simulink model "DuoCopter1"  (R2015b)
settings: Solver=FixedStepAuto  StartTime=0.0  StopTime=150  FixedStep=.01  MaxStep=10  RelTol=1e-3
values from neighbouring files (symbols this model uses):
  AoAMax = 18    [MainDataFile.m]
  RodMass = 1505    [MainDataFile.m]
  s = saveObjectImpl@matlab.System(obj)    [moving_average.m]
undefined symbols (not defined in the file or in its folder): X, Y, Z
libraries: sm_lib x35, Library_Octocopter x19, nesl_utility x17, simulink x3, dspfdesign x1, aerolibfltsims x1
(part 2 of 2)

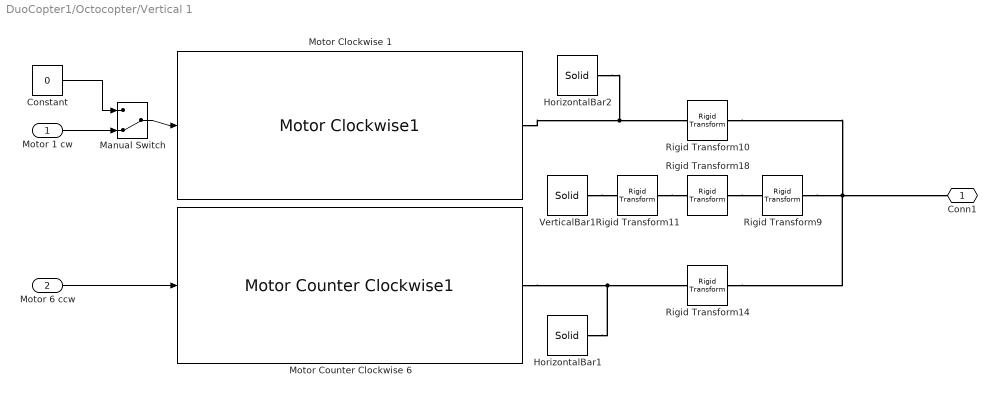
== system DuoCopter1/Octocopter/Vertical 1 ==
  Motor 1 cw : Inport
  Motor 6 ccw : Inport  Port=2
  Constant : Constant  Value=0
  HorizontalBar1 : sm_lib/Body Elements/Solid  InertiaType=PointMass  Mass=462.5  MassUnits=kg  CenterOfMass=[0 0 0]  CenterOfMassUnits=m  MomentsOfInertia=[1 1 1]  MomentsOfInertiaUnits=kg*m^2  ProductsOfInertia=[0 0 0]  ProductsOfInertiaUnits=kg*m^2  DensityBased=on  Density=DensityTube  DensityUnits=kg/(m^3)  DoExposeReferenceFrame=on  SerializedFrames=<Frames/>  GraphicType=FromGeometry  MarkerShape=Sphere  MarkerSize=10  MarkerSizeUnits=m  GraphicVisPropType=SimpleVisualProperties  GraphicDiffuseColor=[0.5 0.5 0.5]  GraphicSpecularColor=[0.5 0.5 0.5 1.0]  GraphicAmbientColor=[0.15 0.15 0.15 1.0]  GraphicEmissiveColor=[0.0 0.0 0.0 1.0]  GraphicShininess=75  GraphicOpacity=1.0  GeometryShape=Sphere  RectangleSize=[1 1]  RectangleSizeUnits=m  BrickDimensions=[1 1 1]  BrickDimensionUnits=m  CylinderRadius=RadiusTube  CylinderRadiusUnits=m  CylinderLength=RodLength  CylinderLengthUnits=m  SphereRadius=.5  SphereRadiusUnits=m  EllipsoidRadii=[1 1 1]  EllipsoidRadiiUnits=m  ExtrusionCrossSection=[1 1; -1 1; -1 -1; 1 -1]  ExtrusionCrossSectionUnits=m  ExtrusionLength=1  ExtrusionLengthUnits=m  PolygonNumSides=3  PolygonOuterRadius=1  PolygonOuterRadiusUnits=m  ExtGeomFileType=STL  ExtGeomFileUnits=m  RevolutionCrossSection=[1 1; 1 -1; 2 -1; 2 1]  RevolutionCrossSectionUnits=m  RevolutionExtent=Full  RevolutionAngle=180  RevolutionAngleUnits=deg  BlockFunction=simmechanics.library.body_elements.solid
  HorizontalBar2 : sm_lib/Body Elements/Solid  InertiaType=PointMass  Mass=462.5  MassUnits=kg  CenterOfMass=[0 0 0]  CenterOfMassUnits=m  MomentsOfInertia=[1 1 1]  MomentsOfInertiaUnits=kg*m^2  ProductsOfInertia=[0 0 0]  ProductsOfInertiaUnits=kg*m^2  DensityBased=on  Density=DensityTube  DensityUnits=kg/(m^3)  DoExposeReferenceFrame=on  SerializedFrames=<Frames/>  GraphicType=FromGeometry  MarkerShape=Sphere  MarkerSize=10  MarkerSizeUnits=m  GraphicVisPropType=SimpleVisualProperties  GraphicDiffuseColor=[0.5 0.5 0.5]  GraphicSpecularColor=[0.5 0.5 0.5 1.0]  GraphicAmbientColor=[0.15 0.15 0.15 1.0]  GraphicEmissiveColor=[0.0 0.0 0.0 1.0]  GraphicShininess=75  GraphicOpacity=1.0  GeometryShape=Sphere  RectangleSize=[1 1]  RectangleSizeUnits=m  BrickDimensions=[1 1 1]  BrickDimensionUnits=m  CylinderRadius=RadiusTube  CylinderRadiusUnits=m  CylinderLength=RodLength  CylinderLengthUnits=m  SphereRadius=.5  SphereRadiusUnits=m  EllipsoidRadii=[1 1 1]  EllipsoidRadiiUnits=m  ExtrusionCrossSection=[1 1; -1 1; -1 -1; 1 -1]  ExtrusionCrossSectionUnits=m  ExtrusionLength=1  ExtrusionLengthUnits=m  PolygonNumSides=3  PolygonOuterRadius=1  PolygonOuterRadiusUnits=m  ExtGeomFileType=STL  ExtGeomFileUnits=m  RevolutionCrossSection=[1 1; 1 -1; 2 -1; 2 1]  RevolutionCrossSectionUnits=m  RevolutionExtent=Full  RevolutionAngle=180  RevolutionAngleUnits=deg  BlockFunction=simmechanics.library.body_elements.solid
  Manual Switch : ManualSwitch  CurrentSetting=0
  Motor Clockwise 1 : Library_Octocopter/Motor Clockwise1
  Motor Counter Clockwise 6 : Library_Octocopter/Motor Counter Clockwise1
  Rigid Transform10 : sm_lib/Frames and Transforms/Rigid Transform  TranslationMethod=Cartesian  TranslationLengthUnit=m  TranslationStandardAxis=+Z  TranslationStandardOffset=0  TranslationCartesianOffset=PositionEngine1  TranslationROffset=0  TranslationROffsetUnits=m  TranslationZOffset=0  TranslationZOffsetUnits=m  TranslationThetaOffset=0  TranslationThetaOffsetUnits=deg  RotationMethod=None  RotationAngleUnits=deg  RotationStandardAxis=+Z  RotationAngle=0  RotationArbitraryAxis=[0 0 1]  FollAlignAxisA=+X  BaseAlignAxisA=+Y  FollAlignAxisB=+Y  BaseAlignAxisB=+Z  RotationSequenceAxes=FollowerAxes  RotationSequence=XYX  RotationSequenceAngles=[0 0 0]  RotationSequenceAnglesUnits=deg  RotationMatrix=[1 0 0; 0 1 0; 0 0 1]  BlockFunction=simmechanics.library.frames_transforms.rigid_transform
  Rigid Transform11 : sm_lib/Frames and Transforms/Rigid Transform  TranslationMethod=Cartesian  TranslationLengthUnit=m  TranslationStandardAxis=+Z  TranslationStandardOffset=0  TranslationCartesianOffset=[0 0 0]  TranslationROffset=0  TranslationROffsetUnits=m  TranslationZOffset=0  TranslationZOffsetUnits=m  TranslationThetaOffset=0  TranslationThetaOffsetUnits=deg  RotationMethod=StandardAxis  RotationAngleUnits=deg  RotationStandardAxis=+Y  RotationAngle=90  RotationArbitraryAxis=[0 0 1]  FollAlignAxisA=+X  BaseAlignAxisA=+Y  FollAlignAxisB=+Y  BaseAlignAxisB=+Z  RotationSequenceAxes=FollowerAxes  RotationSequence=XYX  RotationSequenceAngles=[0 0 0]  RotationSequenceAnglesUnits=deg  RotationMatrix=[1 0 0; 0 1 0; 0 0 1]  BlockFunction=simmechanics.library.frames_transforms.rigid_transform
  Rigid Transform14 : sm_lib/Frames and Transforms/Rigid Transform  TranslationMethod=Cartesian  TranslationLengthUnit=m  TranslationStandardAxis=+Z  TranslationStandardOffset=0  TranslationCartesianOffset=PositionEngine6  TranslationROffset=0  TranslationROffsetUnits=m  TranslationZOffset=0  TranslationZOffsetUnits=m  TranslationThetaOffset=0  TranslationThetaOffsetUnits=deg  RotationMethod=None  RotationAngleUnits=deg  RotationStandardAxis=+Z  RotationAngle=0  RotationArbitraryAxis=[0 0 1]  FollAlignAxisA=+X  BaseAlignAxisA=+Y  FollAlignAxisB=+Y  BaseAlignAxisB=+Z  RotationSequenceAxes=FollowerAxes  RotationSequence=XYX  RotationSequenceAngles=[0 0 0]  RotationSequenceAnglesUnits=deg  RotationMatrix=[1 0 0; 0 1 0; 0 0 1]  BlockFunction=simmechanics.library.frames_transforms.rigid_transform
  Rigid Transform18 : sm_lib/Frames and Transforms/Rigid Transform  TranslationMethod=None  TranslationLengthUnit=m  TranslationStandardAxis=+Z  TranslationStandardOffset=0  TranslationCartesianOffset=[0 0 0]  TranslationROffset=0  TranslationROffsetUnits=m  TranslationZOffset=0  TranslationZOffsetUnits=m  TranslationThetaOffset=0  TranslationThetaOffsetUnits=deg  RotationMethod=StandardAxis  RotationAngleUnits=deg  RotationStandardAxis=+Z  RotationAngle=90  RotationArbitraryAxis=[0 0 1]  FollAlignAxisA=+X  BaseAlignAxisA=+Y  FollAlignAxisB=+Y  BaseAlignAxisB=+Z  RotationSequenceAxes=FollowerAxes  RotationSequence=XYX  RotationSequenceAngles=[0 0 0]  RotationSequenceAnglesUnits=deg  RotationMatrix=[1 0 0; 0 1 0; 0 0 1]  BlockFunction=simmechanics.library.frames_transforms.rigid_transform
  Rigid Transform9 : sm_lib/Frames and Transforms/Rigid Transform  TranslationMethod=Cartesian  TranslationLengthUnit=m  TranslationStandardAxis=+Z  TranslationStandardOffset=0  TranslationCartesianOffset=VerticalBar1  TranslationROffset=0  TranslationROffsetUnits=m  TranslationZOffset=0  TranslationZOffsetUnits=m  TranslationThetaOffset=0  TranslationThetaOffsetUnits=deg  RotationMethod=None  RotationAngleUnits=deg  RotationStandardAxis=+Z  RotationAngle=0  RotationArbitraryAxis=[0 0 1]  FollAlignAxisA=+X  BaseAlignAxisA=+Y  FollAlignAxisB=+Y  BaseAlignAxisB=+Z  RotationSequenceAxes=FollowerAxes  RotationSequence=XYX  RotationSequenceAngles=[0 0 0]  RotationSequenceAnglesUnits=deg  RotationMatrix=[1 0 0; 0 1 0; 0 0 1]  BlockFunction=simmechanics.library.frames_transforms.rigid_transform
  VerticalBar1 : sm_lib/Body Elements/Solid  InertiaType=CalculateFromGeometry  Mass=RodMass  MassUnits=kg  CenterOfMass=[0 0 0]  CenterOfMassUnits=m  MomentsOfInertia=[1 1 1]  MomentsOfInertiaUnits=kg*m^2  ProductsOfInertia=[0 0 0]  ProductsOfInertiaUnits=kg*m^2  DensityBased=off  Density=DensityTube  DensityUnits=kg/(m^3)  DoExposeReferenceFrame=on  SerializedFrames=<Frames/>  GraphicType=FromGeometry  MarkerShape=Sphere  MarkerSize=10  MarkerSizeUnits=m  GraphicVisPropType=SimpleVisualProperties  GraphicDiffuseColor=[0.5 0.5 0.5]  GraphicSpecularColor=[0.5 0.5 0.5 1.0]  GraphicAmbientColor=[0.15 0.15 0.15 1.0]  GraphicEmissiveColor=[0.0 0.0 0.0 1.0]  GraphicShininess=75  GraphicOpacity=1.0  GeometryShape=Cylinder  RectangleSize=[1 1]  RectangleSizeUnits=m  BrickDimensions=[1 1 1]  BrickDimensionUnits=m  CylinderRadius=RadiusTube  CylinderRadiusUnits=m  CylinderLength=RodLength  CylinderLengthUnits=m  SphereRadius=1  SphereRadiusUnits=m  EllipsoidRadii=[1 1 1]  EllipsoidRadiiUnits=m  ExtrusionCrossSection=[1 1; -1 1; -1 -1; 1 -1]  ExtrusionCrossSectionUnits=m  ExtrusionLength=1  ExtrusionLengthUnits=m  PolygonNumSides=3  PolygonOuterRadius=1  PolygonOuterRadiusUnits=m  ExtGeomFileType=STL  ExtGeomFileUnits=m  RevolutionCrossSection=[1 1; 1 -1; 2 -1; 2 1]  RevolutionCrossSectionUnits=m  RevolutionExtent=Full  RevolutionAngle=180  RevolutionAngleUnits=deg  BlockFunction=simmechanics.library.body_elements.solid
  Conn1 : PMIOPort  Port=1  Side=Right
  wires:
  Motor 6 ccw/1 -> Motor Counter Clockwise 6/1
  Constant/1 -> Manual Switch/1
  Motor 1 cw/1 -> Manual Switch/2
  Manual Switch/1 -> Motor Clockwise 1/1
  connections:
  VerticalBar1/RConn1 -- Rigid Transform11/RConn1
  Rigid Transform14/LConn1 -- Conn1/RConn1 -- Rigid Transform10/LConn1 -- Rigid Transform9/LConn1
  Motor Counter Clockwise 6/RConn1 -- HorizontalBar1/RConn1 -- Rigid Transform14/RConn1
  Motor Clockwise 1/RConn1 -- HorizontalBar2/RConn1 -- Rigid Transform10/RConn1
  Rigid Transform11/LConn1 -- Rigid Transform18/RConn1
  Rigid Transform18/LConn1 -- Rigid Transform9/RConn1

== system DuoCopter1/Octocopter/Vertical 2 ==
  "Motor 2 ccw " : Inport
  Motor 5 cw : Inport  Port=2
  HorizontalBar1 : sm_lib/Body Elements/Solid  InertiaType=PointMass  Mass=462.5  MassUnits=kg  CenterOfMass=[0 0 0]  CenterOfMassUnits=m  MomentsOfInertia=[1 1 1]  MomentsOfInertiaUnits=kg*m^2  ProductsOfInertia=[0 0 0]  ProductsOfInertiaUnits=kg*m^2  DensityBased=on  Density=DensityTube  DensityUnits=kg/(m^3)  DoExposeReferenceFrame=on  SerializedFrames=<Frames/>  GraphicType=FromGeometry  MarkerShape=Sphere  MarkerSize=10  MarkerSizeUnits=m  GraphicVisPropType=SimpleVisualProperties  GraphicDiffuseColor=[0.5 0.5 0.5]  GraphicSpecularColor=[0.5 0.5 0.5 1.0]  GraphicAmbientColor=[0.15 0.15 0.15 1.0]  GraphicEmissiveColor=[0.0 0.0 0.0 1.0]  GraphicShininess=75  GraphicOpacity=1.0  GeometryShape=Sphere  RectangleSize=[1 1]  RectangleSizeUnits=m  BrickDimensions=[1 1 1]  BrickDimensionUnits=m  CylinderRadius=RadiusTube  CylinderRadiusUnits=m  CylinderLength=RodLength  CylinderLengthUnits=m  SphereRadius=.5  SphereRadiusUnits=m  EllipsoidRadii=[1 1 1]  EllipsoidRadiiUnits=m  ExtrusionCrossSection=[1 1; -1 1; -1 -1; 1 -1]  ExtrusionCrossSectionUnits=m  ExtrusionLength=1  ExtrusionLengthUnits=m  PolygonNumSides=3  PolygonOuterRadius=1  PolygonOuterRadiusUnits=m  ExtGeomFileType=STL  ExtGeomFileUnits=m  RevolutionCrossSection=[1 1; 1 -1; 2 -1; 2 1]  RevolutionCrossSectionUnits=m  RevolutionExtent=Full  RevolutionAngle=180  RevolutionAngleUnits=deg  BlockFunction=simmechanics.library.body_elements.solid
  HorizontalBar2 : sm_lib/Body Elements/Solid  InertiaType=PointMass  Mass=462.5  MassUnits=kg  CenterOfMass=[0 0 0]  CenterOfMassUnits=m  MomentsOfInertia=[1 1 1]  MomentsOfInertiaUnits=kg*m^2  ProductsOfInertia=[0 0 0]  ProductsOfInertiaUnits=kg*m^2  DensityBased=on  Density=DensityTube  DensityUnits=kg/(m^3)  DoExposeReferenceFrame=on  SerializedFrames=<Frames/>  GraphicType=FromGeometry  MarkerShape=Sphere  MarkerSize=10  MarkerSizeUnits=m  GraphicVisPropType=SimpleVisualProperties  GraphicDiffuseColor=[0.5 0.5 0.5]  GraphicSpecularColor=[0.5 0.5 0.5 1.0]  GraphicAmbientColor=[0.15 0.15 0.15 1.0]  GraphicEmissiveColor=[0.0 0.0 0.0 1.0]  GraphicShininess=75  GraphicOpacity=1.0  GeometryShape=Sphere  RectangleSize=[1 1]  RectangleSizeUnits=m  BrickDimensions=[1 1 1]  BrickDimensionUnits=m  CylinderRadius=RadiusTube  CylinderRadiusUnits=m  CylinderLength=RodLength  CylinderLengthUnits=m  SphereRadius=.5  SphereRadiusUnits=m  EllipsoidRadii=[1 1 1]  EllipsoidRadiiUnits=m  ExtrusionCrossSection=[1 1; -1 1; -1 -1; 1 -1]  ExtrusionCrossSectionUnits=m  ExtrusionLength=1  ExtrusionLengthUnits=m  PolygonNumSides=3  PolygonOuterRadius=1  PolygonOuterRadiusUnits=m  ExtGeomFileType=STL  ExtGeomFileUnits=m  RevolutionCrossSection=[1 1; 1 -1; 2 -1; 2 1]  RevolutionCrossSectionUnits=m  RevolutionExtent=Full  RevolutionAngle=180  RevolutionAngleUnits=deg  BlockFunction=simmechanics.library.body_elements.solid
  Motor Clockwise 5 : Library_Octocopter/Motor Clockwise1
  Motor Counter Clockwise 2 : Library_Octocopter/Motor Counter Clockwise1
  Rigid Transform12 : sm_lib/Frames and Transforms/Rigid Transform  TranslationMethod=Cartesian  TranslationLengthUnit=m  TranslationStandardAxis=+Z  TranslationStandardOffset=0  TranslationCartesianOffset=VerticalBar2  TranslationROffset=0  TranslationROffsetUnits=m  TranslationZOffset=0  TranslationZOffsetUnits=m  TranslationThetaOffset=0  TranslationThetaOffsetUnits=deg  RotationMethod=None  RotationAngleUnits=deg  RotationStandardAxis=+Z  RotationAngle=0  RotationArbitraryAxis=[0 0 1]  FollAlignAxisA=+X  BaseAlignAxisA=+Y  FollAlignAxisB=+Y  BaseAlignAxisB=+Z  RotationSequenceAxes=FollowerAxes  RotationSequence=XYX  RotationSequenceAngles=[0 0 0]  RotationSequenceAnglesUnits=deg  RotationMatrix=[1 0 0; 0 1 0; 0 0 1]  BlockFunction=simmechanics.library.frames_transforms.rigid_transform
  Rigid Transform13 : sm_lib/Frames and Transforms/Rigid Transform  TranslationMethod=Cartesian  TranslationLengthUnit=m  TranslationStandardAxis=+Z  TranslationStandardOffset=0  TranslationCartesianOffset=PositionEngine2  TranslationROffset=0  TranslationROffsetUnits=m  TranslationZOffset=0  TranslationZOffsetUnits=m  TranslationThetaOffset=0  TranslationThetaOffsetUnits=deg  RotationMethod=None  RotationAngleUnits=deg  RotationStandardAxis=+Z  RotationAngle=0  RotationArbitraryAxis=[0 0 1]  FollAlignAxisA=+X  BaseAlignAxisA=+Y  FollAlignAxisB=+Y  BaseAlignAxisB=+Z  RotationSequenceAxes=FollowerAxes  RotationSequence=XYX  RotationSequenceAngles=[0 0 0]  RotationSequenceAnglesUnits=deg  RotationMatrix=[1 0 0; 0 1 0; 0 0 1]  BlockFunction=simmechanics.library.frames_transforms.rigid_transform
  Rigid Transform15 : sm_lib/Frames and Transforms/Rigid Transform  TranslationMethod=Cartesian  TranslationLengthUnit=m  TranslationStandardAxis=+Z  TranslationStandardOffset=0  TranslationCartesianOffset=[0 0 0]  TranslationROffset=0  TranslationROffsetUnits=m  TranslationZOffset=0  TranslationZOffsetUnits=m  TranslationThetaOffset=0  TranslationThetaOffsetUnits=deg  RotationMethod=StandardAxis  RotationAngleUnits=deg  RotationStandardAxis=+Y  RotationAngle=90  RotationArbitraryAxis=[0 0 1]  FollAlignAxisA=+X  BaseAlignAxisA=+Y  FollAlignAxisB=+Y  BaseAlignAxisB=+Z  RotationSequenceAxes=FollowerAxes  RotationSequence=XYX  RotationSequenceAngles=[0 0 0]  RotationSequenceAnglesUnits=deg  RotationMatrix=[1 0 0; 0 1 0; 0 0 1]  BlockFunction=simmechanics.library.frames_transforms.rigid_transform
  Rigid Transform16 : sm_lib/Frames and Transforms/Rigid Transform  TranslationMethod=Cartesian  TranslationLengthUnit=m  TranslationStandardAxis=+Z  TranslationStandardOffset=0  TranslationCartesianOffset=PositionEngine5  TranslationROffset=0  TranslationROffsetUnits=m  TranslationZOffset=0  TranslationZOffsetUnits=m  TranslationThetaOffset=0  TranslationThetaOffsetUnits=deg  RotationMethod=None  RotationAngleUnits=deg  RotationStandardAxis=+Z  RotationAngle=0  RotationArbitraryAxis=[0 0 1]  FollAlignAxisA=+X  BaseAlignAxisA=+Y  FollAlignAxisB=+Y  BaseAlignAxisB=+Z  RotationSequenceAxes=FollowerAxes  RotationSequence=XYX  RotationSequenceAngles=[0 0 0]  RotationSequenceAnglesUnits=deg  RotationMatrix=[1 0 0; 0 1 0; 0 0 1]  BlockFunction=simmechanics.library.frames_transforms.rigid_transform
  Rigid Transform17 : sm_lib/Frames and Transforms/Rigid Transform  TranslationMethod=None  TranslationLengthUnit=m  TranslationStandardAxis=+Z  TranslationStandardOffset=0  TranslationCartesianOffset=[0 0 0]  TranslationROffset=0  TranslationROffsetUnits=m  TranslationZOffset=0  TranslationZOffsetUnits=m  TranslationThetaOffset=0  TranslationThetaOffsetUnits=deg  RotationMethod=StandardAxis  RotationAngleUnits=deg  RotationStandardAxis=+Z  RotationAngle=90  RotationArbitraryAxis=[0 0 1]  FollAlignAxisA=+X  BaseAlignAxisA=+Y  FollAlignAxisB=+Y  BaseAlignAxisB=+Z  RotationSequenceAxes=FollowerAxes  RotationSequence=XYX  RotationSequenceAngles=[0 0 0]  RotationSequenceAnglesUnits=deg  RotationMatrix=[1 0 0; 0 1 0; 0 0 1]  BlockFunction=simmechanics.library.frames_transforms.rigid_transform
  VerticalBar 2 : sm_lib/Body Elements/Solid  InertiaType=CalculateFromGeometry  Mass=RodMass  MassUnits=kg  CenterOfMass=[0 0 0]  CenterOfMassUnits=m  MomentsOfInertia=[1 1 1]  MomentsOfInertiaUnits=kg*m^2  ProductsOfInertia=[0 0 0]  ProductsOfInertiaUnits=kg*m^2  DensityBased=off  Density=DensityTube  DensityUnits=kg/(m^3)  DoExposeReferenceFrame=on  SerializedFrames=<Frames/>  GraphicType=FromGeometry  MarkerShape=Sphere  MarkerSize=10  MarkerSizeUnits=m  GraphicVisPropType=SimpleVisualProperties  GraphicDiffuseColor=[0.5 0.5 0.5]  GraphicSpecularColor=[0.5 0.5 0.5 1.0]  GraphicAmbientColor=[0.15 0.15 0.15 1.0]  GraphicEmissiveColor=[0.0 0.0 0.0 1.0]  GraphicShininess=75  GraphicOpacity=1.0  GeometryShape=Cylinder  RectangleSize=[1 1]  RectangleSizeUnits=m  BrickDimensions=[1 1 1]  BrickDimensionUnits=m  CylinderRadius=RadiusTube  CylinderRadiusUnits=m  CylinderLength=RodLength  CylinderLengthUnits=m  SphereRadius=1  SphereRadiusUnits=m  EllipsoidRadii=[1 1 1]  EllipsoidRadiiUnits=m  ExtrusionCrossSection=[1 1; -1 1; -1 -1; 1 -1]  ExtrusionCrossSectionUnits=m  ExtrusionLength=1  ExtrusionLengthUnits=m  PolygonNumSides=3  PolygonOuterRadius=1  PolygonOuterRadiusUnits=m  ExtGeomFileType=STL  ExtGeomFileUnits=m  RevolutionCrossSection=[1 1; 1 -1; 2 -1; 2 1]  RevolutionCrossSectionUnits=m  RevolutionExtent=Full  RevolutionAngle=180  RevolutionAngleUnits=deg  BlockFunction=simmechanics.library.body_elements.solid
  Conn1 : PMIOPort  Port=1  Side=Right
  wires:
  Motor 5 cw/1 -> Motor Clockwise 5/1
  "Motor 2 ccw "/1 -> Motor Counter Clockwise 2/1
  connections:
  VerticalBar 2/RConn1 -- Rigid Transform15/RConn1
  Rigid Transform17/RConn1 -- Rigid Transform15/LConn1
  Rigid Transform17/LConn1 -- Rigid Transform12/RConn1
  Rigid Transform16/LConn1 -- Conn1/RConn1 -- Rigid Transform13/LConn1 -- Rigid Transform12/LConn1
  Motor Counter Clockwise 2/RConn1 -- HorizontalBar2/RConn1 -- Rigid Transform13/RConn1
  Motor Clockwise 5/RConn1 -- HorizontalBar1/RConn1 -- Rigid Transform16/RConn1

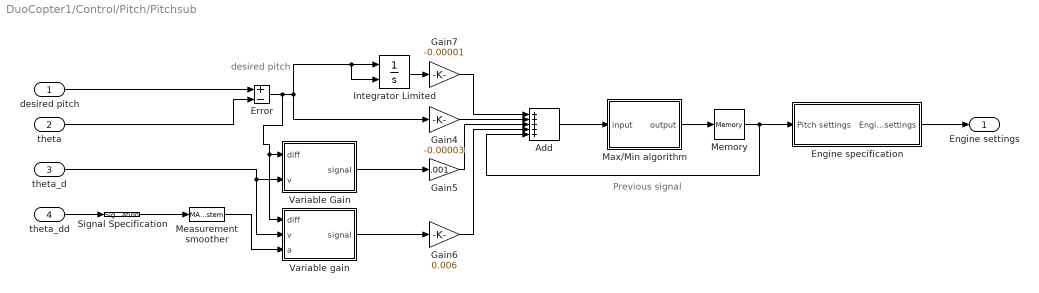
== system DuoCopter1/Control/Pitch/Pitchsub ==
  note: Previous signal
  note: desired pitch
  desired pitch : Inport
  theta : Inport  Port=2
  theta_d : Inport  Port=3
  theta_dd : Inport  Port=4
  Add : Sum  Inputs=+++++
  Engine specification : Subsystem
  Error : Sum  Inputs=+-
  Gain4 : Gain  Gain=-0.00003
  Gain5 : Gain  Gain=.001
  Gain6 : Gain  Gain=0.006
  Gain7 : Gain  Gain=-0.00001
  Integrator Limited : Integrator  ExternalReset=either  LimitOutput=on  UpperSaturationLimit=1  LowerSaturationLimit=-1
  Max/Min algorithm : MATLAB Function  TreatAsAtomicUnit=on
  Measurement smoother : MATLABSystem  System=moving_average  WindowLength=1  SimulateUsing=Interpreted execution
      mask Type: moving_average
      mask Display:
      | disp('moving_average');
      | port_label('input',1,'X');
      | port_label('output',1,'Y');
  Memory : Memory  InheritSampleTime=on  LinearizeAsDelay=on
  Signal Specification : SignalSpecification  Dimensions=1
  Variable Gain : MATLAB Function  TreatAsAtomicUnit=on
  Variable gain : MATLAB Function  TreatAsAtomicUnit=on
  Engine settings : Outport
  wires:
  theta/1 -> Error/2
  desired pitch/1 -> Error/1
  Integrator Limited/1 -> Gain7/1
  Error/1 -> Variable gain/1(diff), Variable Gain/1(diff), Integrator Limited/2, Integrator Limited/1, Gain4/1
  Gain4/1 -> Add/2
  Gain5/1 -> Add/3
  Add/1 -> Max/Min algorithm/1(input)
  Gain7/1 -> Add/1
  theta_dd/1 -> Signal Specification/1
  Gain6/1 -> Add/4
  Signal Specification/1 -> Measurement smoother/1
  Memory/1 -> Add/5, Engine specification/1(Pitch settings)
  theta_d/1 -> Variable gain/2(v), Variable Gain/2(v)
  Variable Gain/1(signal) -> Gain5/1
  Measurement smoother/1 -> Variable gain/3(a)
  Variable gain/1(signal) -> Gain6/1
  Max/Min algorithm/1(output) -> Memory/1
  Engine specification/1(Engine settings) -> Engine settings/1

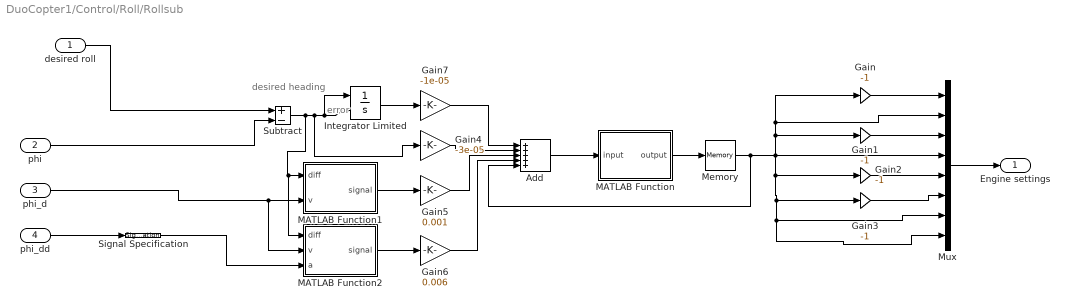
== system DuoCopter1/Control/Roll/Rollsub ==
  note: desired heading
  note: error
  desired roll : Inport
  phi : Inport  Port=2
  phi_d : Inport  Port=3
  phi_dd : Inport  Port=4
  Add : Sum  Inputs=+++++
  Gain{,1..3} (4 alike) : Gain  Gain=-1
  Gain4 : Gain  Gain=-3e-05
  Gain5 : Gain  Gain=0.001
  Gain6 : Gain  Gain=0.006
  Gain7 : Gain  Gain=-1e-05
  Integrator Limited : Integrator  ExternalReset=either  LimitOutput=on  UpperSaturationLimit=1  LowerSaturationLimit=-1
  MATLAB Function : MATLAB Function  TreatAsAtomicUnit=on
  MATLAB Function1 : MATLAB Function  TreatAsAtomicUnit=on
  MATLAB Function2 : MATLAB Function  TreatAsAtomicUnit=on
  Memory : Memory  InheritSampleTime=on  LinearizeAsDelay=on
  Mux : Mux  Inputs=8
  Signal Specification : SignalSpecification  Dimensions=1
  Subtract : Sum  Inputs=+-
  Engine settings : Outport
  wires:
  phi/1 -> Subtract/2
  desired roll/1 -> Subtract/1
  Mux/1 -> Engine settings/1
  Gain/1 -> Mux/1
  Gain2/1 -> Mux/5
  Gain1/1 -> Mux/3
  Gain3/1 -> Mux/6
  phi_dd/1 -> Signal Specification/1
  Integrator Limited/1 -> Gain7/1
  Subtract/1 -> MATLAB Function2/1(diff), MATLAB Function1/1(diff), Gain4/1, Integrator Limited/1, Integrator Limited/2
  Gain4/1 -> Add/2
  Gain5/1 -> Add/3
  Add/1 -> MATLAB Function/1(input)
  Gain7/1 -> Add/1
  Gain6/1 -> Add/4
  Memory/1 -> Add/5, Gain/1, Mux/2, Gain1/1, Gain2/1, Mux/8, Mux/7, Gain3/1, Mux/4
  MATLAB Function1/1(signal) -> Gain5/1
  phi_d/1 -> MATLAB Function1/2(v), MATLAB Function2/2(v)
  Signal Specification/1 -> MATLAB Function2/3(a)
  MATLAB Function2/1(signal) -> Gain6/1
  MATLAB Function/1(output) -> Memory/1

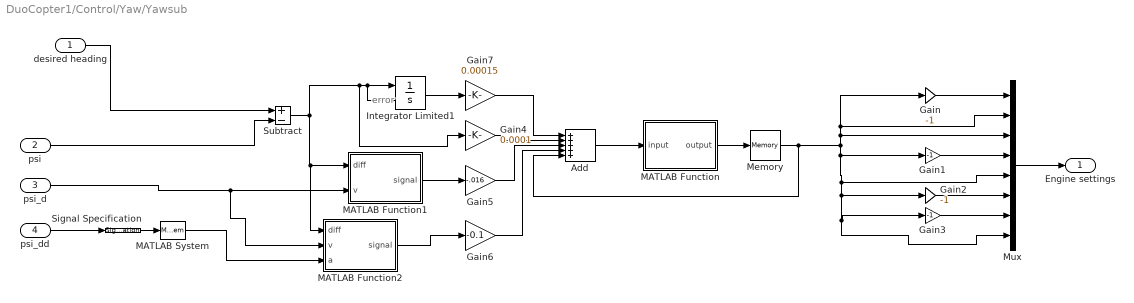
== system DuoCopter1/Control/Yaw/Yawsub ==
  note: error
  desired heading : Inport
  psi : Inport  Port=2
  psi_d : Inport  Port=3
  psi_dd : Inport  Port=4
  Add : Sum  Inputs=+++++
  Gain{,1..3} (4 alike) : Gain  Gain=-1
  Gain4 : Gain  Gain=0.0001
  Gain5 : Gain  Gain=-.016
  Gain6 : Gain  Gain=-0.1
  Gain7 : Gain  Gain=0.00015
  Integrator Limited1 : Integrator  ExternalReset=either  LimitOutput=on  UpperSaturationLimit=1  LowerSaturationLimit=-1
  MATLAB Function : MATLAB Function  TreatAsAtomicUnit=on
  MATLAB Function1 : MATLAB Function  TreatAsAtomicUnit=on
  MATLAB Function2 : MATLAB Function  TreatAsAtomicUnit=on
  MATLAB System : MATLABSystem  System=moving_average  WindowLength=1  SimulateUsing=Interpreted execution
      mask Type: moving_average
      mask Display:
      | disp('moving_average');
      | port_label('input',1,'X');
      | port_label('output',1,'Y');
  Memory : Memory  InheritSampleTime=on  LinearizeAsDelay=on
  Mux : Mux  Inputs=8
  Signal Specification : SignalSpecification  Dimensions=1
  Subtract : Sum  Inputs=+-
  Engine settings : Outport
  wires:
  Gain2/1 -> Mux/6
  psi/1 -> Subtract/2
  desired heading/1 -> Subtract/1
  psi_d/1 -> MATLAB Function2/2(v), MATLAB Function1/2(v)
  Mux/1 -> Engine settings/1
  Gain/1 -> Mux/1
  Gain1/1 -> Mux/4
  Gain3/1 -> Mux/7
  psi_dd/1 -> Signal Specification/1
  Signal Specification/1 -> MATLAB System/1
  Integrator Limited1/1 -> Gain7/1
  Subtract/1 -> MATLAB Function2/1(diff), MATLAB Function1/1(diff), Gain4/1, Integrator Limited1/2, Integrator Limited1/1
  Gain4/1 -> Add/2
  Gain5/1 -> Add/3
  Add/1 -> MATLAB Function/1(input)
  Gain7/1 -> Add/1
  Gain6/1 -> Add/4
  Memory/1 -> Add/5, Mux/5, Gain3/1, Mux/8, Gain2/1, Gain1/1, Mux/2, Gain/1, Mux/3
  MATLAB Function1/1(signal) -> Gain5/1
  MATLAB System/1 -> MATLAB Function2/3(a)
  MATLAB Function/1(output) -> Memory/1
  MATLAB Function2/1(signal) -> Gain6/1

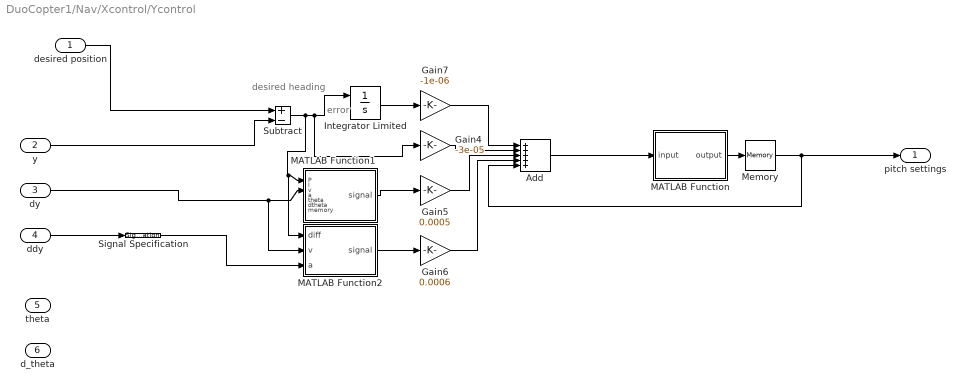
== system DuoCopter1/Nav/Xcontrol/Ycontrol ==
  note: desired heading
  note: error
  desired position : Inport
  y : Inport  Port=2
  dy : Inport  Port=3
  ddy : Inport  Port=4
  theta : Inport  Port=5
  d_theta : Inport  Port=6
  Add : Sum  Inputs=+++++
  Gain4 : Gain  Gain=-3e-05
  Gain5 : Gain  Gain=0.0005
  Gain6 : Gain  Gain=0.0006
  Gain7 : Gain  Gain=-1e-06
  Integrator Limited : Integrator  ExternalReset=either  LimitOutput=on  UpperSaturationLimit=10  LowerSaturationLimit=-10
  MATLAB Function : MATLAB Function  TreatAsAtomicUnit=on
  MATLAB Function1 : MATLAB Function  TreatAsAtomicUnit=on
  MATLAB Function2 : MATLAB Function  TreatAsAtomicUnit=on
  Memory : Memory  InheritSampleTime=on  LinearizeAsDelay=on
  Signal Specification : SignalSpecification  Dimensions=1
  Subtract : Sum  Inputs=+-
  pitch settings : Outport
  wires:
  y/1 -> Subtract/2
  desired position/1 -> Subtract/1
  ddy/1 -> Signal Specification/1
  Integrator Limited/1 -> Gain7/1
  Subtract/1 -> MATLAB Function2/1(diff), MATLAB Function1/1(P), Gain4/1, Integrator Limited/1
  Gain4/1 -> Add/2
  Gain5/1 -> Add/3
  Gain7/1 -> Add/1
  Gain6/1 -> Add/4
  Memory/1 -> Add/5, pitch settings/1
  MATLAB Function1/1(signal) -> Gain5/1
  dy/1 -> MATLAB Function1/3(v), MATLAB Function2/2(v)
  Signal Specification/1 -> MATLAB Function2/3(a)
  MATLAB Function2/1(signal) -> Gain6/1
  MATLAB Function/1(output) -> Memory/1
  Add/1 -> MATLAB Function/1(input)

== system DuoCopter1/Octocopter/6 DOF joint/Subsystem ==
  In1 : Inport
  Demux : Demux  Outputs=3
  Demux1 : Demux  Outputs=2
  MATLAB Function : MATLAB Function  TreatAsAtomicUnit=on
  MATLAB Function1 : MATLAB Function  TreatAsAtomicUnit=on
  MATLAB Function2 : MATLAB Function  TreatAsAtomicUnit=on
  Mux : Mux  Inputs=3
  Out1 : Outport
  wires:
  In1/1 -> Demux/1
  Mux/1 -> Out1/1
  Demux/2 -> MATLAB Function1/1(u)
  Demux/3 -> MATLAB Function2/1(u)
  MATLAB Function/1(y) -> Mux/1
  Demux/1 -> Demux1/1
  Demux1/2 -> MATLAB Function/1(u)
  MATLAB Function1/1(y) -> Mux/2
  MATLAB Function2/1(y) -> Mux/3

== system DuoCopter1/Control/Pitch/Pitchsub/Engine specification ==
  Pitch settings : Inport
  Gain{,1..3} (4 alike) : Gain  Gain=-1
  Mux : Mux  Inputs=8
  Engine settings : Outport
  wires:
  Pitch settings/1 -> Gain2/1, Mux/6, Gain3/1, Mux/8, Mux/4, Gain/1, Gain1/1, Mux/3
  Mux/1 -> Engine settings/1
  Gain/1 -> Mux/1
  Gain3/1 -> Mux/7
  Gain2/1 -> Mux/5
  Gain1/1 -> Mux/2

== matlab function DuoCopter1/Control/Yaw/Yawsub/MATLAB Function ==
  data: input input; output output
function output   = maximum(input)
     if input > 0.5
            output = 0.5;
        elseif input < -0.5
            output = -0.5;
        else
            output = input;
        end
end

== matlab function DuoCopter1/Control/Altitude/MATLAB Function ==
  data: input input; output output
function output   = maximum(input)
     if input > 0.9
            output = 0.9;
        elseif input < 0.3
            output = 0.3;
        else
            output = input;
        end
end

== matlab function DuoCopter1/Control/Pitch/Pitchsub/Max//Min algorithm ==
  data: input input; output output
function output   = maximum(input)
     if input > 0.5
            output = 0.5;
        elseif input < -0.5
            output = -0.5;
        else
            output = input;
        end
end

== matlab function DuoCopter1/Control/Roll/Rollsub/MATLAB Function ==
  data: input input; output output
function output   = maximum(input)
     if input > 0.5
            output = 0.5;
        elseif input < -0.5
            output = -0.5;
        else
            output = input;
        end
end

== matlab function DuoCopter1/Control/MinMax/MATLAB Function ==
  data: input input; output output
function output   = maximum(input)
     if input > 1
            output = 1;
        elseif input < 0
            output = 0;
        else
            output = input;
        end
end

== matlab function DuoCopter1/Control/MinMax/MATLAB Function1 ==
  data: input input; output output
function output   = maximum(input)
     if input > 1
            output = 1;
        elseif input < 0
            output = 0;
        else
            output = input;
        end
end

== matlab function DuoCopter1/Control/MinMax/MATLAB Function2 ==
  data: input input; output output
function output   = maximum(input)
     if input > 1
            output = 1;
        elseif input < 0
            output = 0;
        else
            output = input;
        end
end

== matlab function DuoCopter1/Control/MinMax/MATLAB Function3 ==
  data: input input; output output
function output   = maximum(input)
     if input > 1
            output = 1;
        elseif input < 0
            output = 0;
        else
            output = input;
        end
end

== matlab function DuoCopter1/Control/MinMax/MATLAB Function4 ==
  data: input input; output output
function output   = maximum(input)
     if input > 1
            output = 1;
        elseif input < 0
            output = 0;
        else
            output = input;
        end
end

== matlab function DuoCopter1/Control/MinMax/MATLAB Function5 ==
  data: input input; output output
function output   = maximum(input)
     if input > 1
            output = 1;
        elseif input < 0
            output = 0;
        else
            output = input;
        end
end

== matlab function DuoCopter1/Control/MinMax/MATLAB Function6 ==
  data: input input; output output
function output   = maximum(input)
     if input > 1
            output = 1;
        elseif input < 0
            output = 0;
        else
            output = input;
        end
end

== matlab function DuoCopter1/Control/MinMax/MATLAB Function7 ==
  data: input input; output output
function output   = maximum(input)
     if input > 1
            output = 1;
        elseif input < 0
            output = 0;
        else
            output = input;
        end
end

== matlab function DuoCopter1/Octocopter/6 DOF joint/Subsystem/MATLAB Function ==
  data: u input; y output
function y = fcn(u)

y = real(2*asin(complex(u)));

== matlab function DuoCopter1/Octocopter/6 DOF joint/Subsystem/MATLAB Function1 ==
  data: u input; y output
function y = fcn(u)

y = real(2*asin(complex(u)));

== matlab function DuoCopter1/Octocopter/6 DOF joint/Subsystem/MATLAB Function2 ==
  data: u input; y output
function y = fcn(u)

y = real(2*asin(complex(u)));

== matlab function DuoCopter1/Atmosphere/MATLAB Function ==
  data: u input; y output
function y = fcn(u)
%#codegen

y = -0.0001 .* u + 1.2159;;

== matlab function DuoCopter1/Control/Altitude/MATLAB Function1 ==
  data: diff input; signal output; v input
function signal   = vfilter( diff, v )
if diff/v<0
    signal = 4*v;
elseif diff/v <1
    signal = 1.5*v;
elseif diff <= 15
    signal = v;
elseif diff/v >=1 && diff/v <= 4
        signal = v;
elseif diff/v >=4 && diff/v <=10
    signal = 0.75 * v;
else
    signal = 0;
end

== matlab function DuoCopter1/Control/Altitude/MATLAB Function2 ==
  data: diff input; signal output; v input; a input
function signal   = vfilter( diff, v, a )
if diff/v > 20
    signal = 0;
elseif diff/v < 0
    signal = 0.1 *a;
elseif abs(a)>1
    signal = 10 * a;
elseif abs(a)>0.5
    signal = 4*a;
elseif abs(a)>0.2
    signal = 2*a;
else
    signal = a;
end

== matlab function DuoCopter1/Nav/MATLAB Function ==
  data: input input; output output
function output   = maximum(input)
     if input > 1
            output = 1;
        elseif input < 0
            output = 0;
        else
            output = input;
        end
end

== matlab function DuoCopter1/Control/Pitch/Pitchsub/Variable Gain ==
  data: diff input; signal output; v input
function signal   = vfilter( diff, v )
if diff/v < 0
    signal = 4*v;
elseif diff/v <1
    signal = 2*v;
elseif diff <= .03
    signal = v;
elseif diff/v >=1 && diff/v <= 4
        signal = v;
elseif diff/v >=4 && diff/v <=10
    signal = 0.75 * v;
else
    signal = 0;
end

== matlab function DuoCopter1/Control/Roll/Rollsub/MATLAB Function1 ==
  data: diff input; signal output; v input
function signal   = vfilter( diff, v )
if diff/v < 0
    signal = 4*v;
elseif diff/v <1
    signal = 1.5*v;
elseif diff <= .03
    signal = v;
elseif diff/v >=1 && diff/v <= 4
        signal = v;
elseif diff/v >=4 && diff/v <=10
    signal = 0.75 * v;
else
    signal = 0;
end

== matlab function DuoCopter1/Control/Yaw/Yawsub/MATLAB Function1 ==
  data: diff input; signal output; v input
function signal   = vfilter( diff, v )
if diff/v <0
    signal = 7*v;
elseif diff/v <2
    signal = 2*v;
elseif diff/v >=2 && diff/v <= 6
        signal = 1.5*v;
elseif diff/v >=6 && diff/v <=10
    signal = 0.75 * v;
else
    signal = 0;
end

== matlab function DuoCopter1/Control/Yaw/Yawsub/MATLAB Function2 ==
  data: diff input; signal output; v input; a input
function signal   = vfilter( diff, v, a )
if diff/v > 20
    signal = 0;
elseif diff/v < 0
    signal = 0.2*a;
elseif abs(a)>1
    signal = 10 * a;
elseif abs(a)>0.5
    signal = 4*a;
elseif abs(a)>0.2
    signal = 2*a
else
    signal = a;
end

== matlab function DuoCopter1/Control/Pitch/Pitchsub/Variable gain ==
  data: diff input; signal output; v input; a input
function signal   = vfilter( diff, v, a )
if diff/v > 20
    signal = 0;
elseif diff/v < 0
    signal = 0.4 *a;
elseif abs(a)>1
    signal = 10 * a;
elseif abs(a)>0.5
    signal = 4*a;
elseif abs(a)>0.2
    signal = 2*a;
else
    signal = a;
end

== matlab function DuoCopter1/Control/Roll/Rollsub/MATLAB Function2 ==
  data: diff input; signal output; v input; a input
function signal   = vfilter( diff, v, a )
if diff/v > 20
    signal = 0;
elseif diff/v < 0
    signal = 0.1 *a;
elseif abs(a)>1
    signal = 10 * a;
elseif abs(a)>0.5
    signal = 4*a;
elseif abs(a)>0.2
    signal = 2*a;
else
    signal = a;
end

== matlab function DuoCopter1/Nav/Xcontrol/Ycontrol/MATLAB Function ==
  data: input input; output output
function output   = maximum(input)
     if input > pi/8
            output = pi/8;
        elseif input < -pi/8
            output = -pi/8;
        else
            output = input;
        end
end

== matlab function DuoCopter1/Nav/Xcontrol/Ycontrol/MATLAB Function1 ==
  data: P input; I input; signal output; v input; a input; theta input; dtheta input; memory input
function signal   = vfilter( P, I, v, a, theta, dtheta, memory )
T = P/v
Treq = theta 





signal = v
end

== matlab function DuoCopter1/Nav/Xcontrol/Ycontrol/MATLAB Function2 ==
  data: diff input; signal output; v input; a input
function signal   = vfilter( diff, v, a )
if diff/v > 20
    signal = 0;
elseif diff/v < 0
    signal = 0.1 *a;
elseif abs(a)>1
    signal = 10 * a;
elseif abs(a)>0.5
    signal = 4*a;
elseif abs(a)>0.2
    signal = 2*a;
else
    signal = a;
end
